simulink model "Racing_2019"  (R2017a)
settings: Solver=FixedStepDiscrete  StartTime=0.0  StopTime=Inf  FixedStep=1e-3  RelTol=1e-3  EnableMultiTasking=on
PostLoadFcn:
  | , if any(exist('dsrtsu_mdlpostloadfcn', 'file') == [2, 3, 6]), try dsrtsu_mdlpostloadfcn('Execute', bdroot); catch fprintf('Error in PostLoadFcn (dsrtsu_mdlpostloadfcn) for model "%s":\n %s\n', bdroot, lasterr); end, end,
undefined symbols (not defined in the file): Accu_Fans_Enable, Accu_Fans_ON, Accu_Fans_PWM, APPS_Bypass, APPS_Value, AUX_Error_Time, Batt_Temp_High_Threshold, Batt_Temp_Low_Threshold, BMS_Error_Time, BMS_Reset, BMS_Reset_Enable, BMS_Status_Bypass, Brake_Plausibility_Threshold, Brake_Threshold, Brakelight_Test, Braking_Torque, BSPD_State_Bypass, Buzzer, Buzzer_Silent, Buzzer_Test, Calibrate, CAN_Rx_FMEA_Enable, CAN_Status_FMEA_Enable, CAN_Tx_FMEA_Enable, Car_Reset, Car_Reset_Enable, Dash_Fan_PWM, DiscIntNeverNeededParam, DRS_Enable, DRS_PWM_OFF, DRS_PWM_ON, ED_Enable, ED_On, Eject_USB, Enable_Kill, Enable_LED_Test, Fans_Left_Enable, Fans_Left_ON, Fans_Left_PWM, Fans_Right_Enable, Fans_Right_ON, Fans_Right_PWM, I_MAX, IGBT_Temp_High_Threshold, IGBT_Temp_Low_Threshold, Inverter_CAN_Tx_Enable, Inverter_Frequency, KW_Max_Regen_Reset, KW_Max_Reset, LV_DCDC_Temp_High_Threshold, LV_DCDC_Temp_Low_Threshold, magnitude, Plausibility_Bypass, Power_Limiter_Killswitch, Power_Target_kW, Pump_Left_Enable, Pump_Left_ON, Pump_Right_Enable, Pump_Right_ON, Pump_Signal_Left ... (+13)
libraries: rtiusbflightreclib x206, simulink x153, rtican x52, powerlib_meascontrol x47, simulink_extras x17, rti1401lib_adc_type4 x6, rti1401lib_dio_type4 x3, rti1401lib_II_base x1
(part 9 of 23)

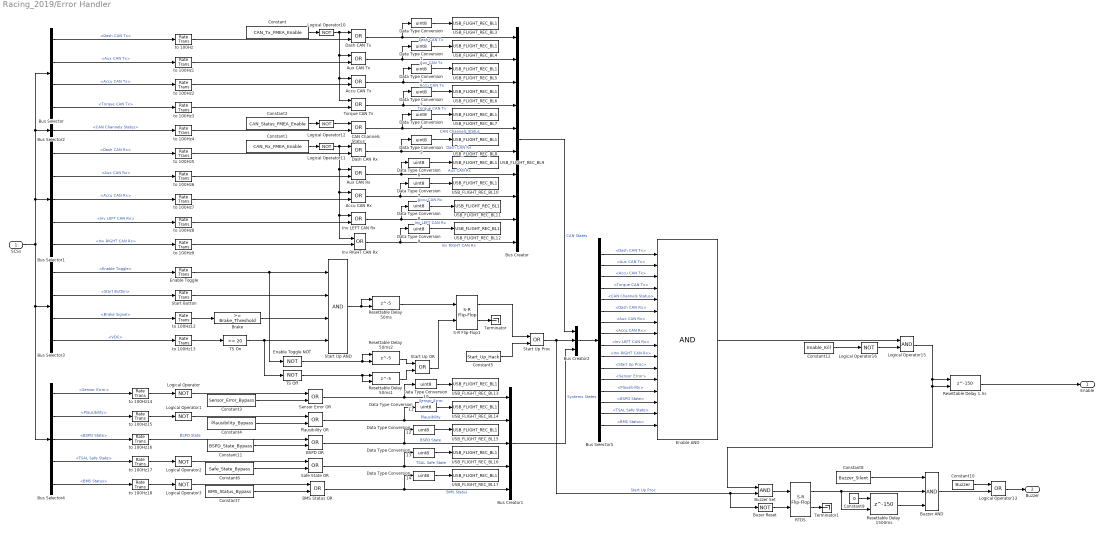
== system Racing_2019/Error Handler ==
  SCSs : Inport
  Accu CAN Rx : Logic  Operator=OR  AllPortsSameDT=off  OutDataTypeStr=boolean
  Accu CAN Tx : Logic  Operator=OR  AllPortsSameDT=off  OutDataTypeStr=boolean
  Aux CAN Rx : Logic  Operator=OR  AllPortsSameDT=off  OutDataTypeStr=boolean
  Aux CAN Tx : Logic  Operator=OR  AllPortsSameDT=off  OutDataTypeStr=boolean
  BMS Status OR : Logic  Operator=OR  AllPortsSameDT=off  OutDataTypeStr=boolean
  BSPD OR : Logic  Operator=OR  AllPortsSameDT=off  OutDataTypeStr=boolean
  Brake : simulink/Logic and Bit Operations/Compare To Constant  relop=>=  const=Brake_Threshold  OutDataTypeStr=boolean
  Bus Creator : BusCreator  Inputs='Dash CAN Tx','Aux CAN Tx','Accu CAN Tx','Torque CAN Tx','CAN Channels Status','Dash CAN Rx','Aux CAN Rx','Accu CAN Rx','Inv LEFT CAN Rx','Inv RIGHT CAN Rx'
  Bus Creator1 : BusCreator  Inputs='Sensor Error','Plausibility','BSPD State','TSAL Safe State','BMS Status'
  Bus Creator2 : BusCreator  Inputs=3
  Bus Selector : BusSelector  OutputSignals=Error & Feedback.CAN Tx Feedback.Dash CAN Tx,Error & Feedback.CAN Tx Feedback.Aux CAN Tx,Error & Feedback.CAN Tx Feedback.Accu CAN Tx,Error & Feedback.CAN Tx Feedback.Torque CAN Tx
  Bus Selector1 : BusSelector  OutputSignals=Inputs.from Dashboard.Dash CAN Rx,Inputs.from Aux.Aux CAN Rx,Inputs.from Accu.Accu CAN Rx,Inputs.from Inv LEFT.Inv LEFT CAN Rx,Inputs.from Inv RIGHT.Inv RIGHT CAN Rx
  Bus Selector2 : BusSelector  OutputSignals=Inputs.CAN Channels Status
  Bus Selector3 : BusSelector  OutputSignals=Inputs.from Dashboard.Enable Toggle,Inputs.from Dashboard.Start Button,Inputs.from Dashboard.Brake Signal,Inputs.from Gen Inputs.VDC
  Bus Selector4 : BusSelector  OutputSignals=Error & Feedback.Sensor Error,Error & Feedback.Plausibility,Inputs.from Aux.BSPD State,Inputs.from Aux.TSAL Safe State,Inputs.from Accu.BMS Status
  Bus Selector5 : BusSelector  OutputSignals=CAN States.Dash CAN Tx,CAN States.Aux CAN Tx,CAN States.Accu CAN Tx,CAN States.Torque CAN Tx,CAN States.CAN Channels Status,CAN States.Dash CAN Rx,CAN States.Aux CAN Rx,CAN States.Accu CAN Rx,CAN States.Inv LEFT CAN Rx,CAN States.Inv RIGHT CAN Rx,Start Up Proc,Systems States.Sensor Error,Systems States.Plausibility,Systems States.BSPD State,Systems States.TSAL Safe State,Systems States.BMS Status
  Buzer Reset : Logic  Operator=NOT  AllPortsSameDT=off  OutDataTypeStr=boolean
  Buzzer AND : Logic  Inputs=3  AllPortsSameDT=off  OutDataTypeStr=boolean
  Buzzer Set : Logic  AllPortsSameDT=off  OutDataTypeStr=boolean
  CAN Channels Status : Logic  Operator=OR  AllPortsSameDT=off  OutDataTypeStr=boolean
  Constant : Constant  Value=CAN_Tx_FMEA_Enable
  Constant1 : Constant  Value=CAN_Rx_FMEA_Enable
  Constant10 : Constant  Value=Buzzer
  Constant11 : Constant  Value=BSPD_State_Bypass
  Constant12 : Constant  Value=Enable_Kill
  Constant2 : Constant  Value=CAN_Status_FMEA_Enable
  Constant3 : Constant  Value=Sensor_Error_Bypass
  Constant4 : Constant  Value=Plausibility_Bypass
  Constant5 : Constant  Value=Start_Up_Hack
  Constant6 : Constant  Value=Safe_State_Bypass
  Constant7 : Constant  Value=BMS_Status_Bypass
  Constant8 : Constant  Value=Buzzer_Silent
  Constant9 : Constant  Value=0
  Dash CAN Rx : Logic  Operator=OR  AllPortsSameDT=off  OutDataTypeStr=boolean
  Dash CAN Tx : Logic  Operator=OR  AllPortsSameDT=off  OutDataTypeStr=boolean
  Data Type Conversion{,1..14} (15 alike) : DataTypeConversion  OutDataTypeStr=uint8
  Enable AND : Logic  Inputs=16  AllPortsSameDT=off  OutDataTypeStr=boolean
  Enable Toggle : RateTransition  OutPortSampleTime=0.01
  Enable Toggle NOT : Logic  Operator=NOT  AllPortsSameDT=off  OutDataTypeStr=boolean
  Inv LEFT CAN Rx : Logic  Operator=OR  AllPortsSameDT=off  OutDataTypeStr=boolean
  Inv RIGHT CAN Rx : Logic  Operator=OR  AllPortsSameDT=off  OutDataTypeStr=boolean
  Logical Operator{,1..3,10..12,16} (8 alike) : Logic  Operator=NOT  AllPortsSameDT=off  OutDataTypeStr=boolean
  Logical Operator13 : Logic  Operator=OR  AllPortsSameDT=off  OutDataTypeStr=boolean
  Logical Operator15 : Logic  AllPortsSameDT=off  OutDataTypeStr=boolean
  Plausibility OR : Logic  Operator=OR  AllPortsSameDT=off  OutDataTypeStr=boolean
  RTDS : simulink_extras/Flip Flops/S-R Flip-Flop  initial_condition=0
  Resettable Delay 1.5s : Delay  DelayLength=150  ExternalReset=Falling
      settings: InputPortMap=u0,r5
  Resettable Delay 1500ms : Delay  DelayLength=150  InitialCondition=1  ExternalReset=Rising
      settings: InputPortMap=u0,r5
  Resettable Delay 50ms : Delay  DelayLength=5  ExternalReset=Falling
      settings: InputPortMap=u0,r5
  Resettable Delay 50ms1 : Delay  DelayLength=5  InitialCondition=1  ExternalReset=Rising
      settings: InputPortMap=u0,r5
  Resettable Delay 50ms2 : Delay  DelayLength=5  InitialCondition=1  ExternalReset=Rising
      settings: InputPortMap=u0,r5
  S-R Flip-Flop1 : simulink_extras/Flip Flops/S-R Flip-Flop  initial_condition=0
  Safe State OR : Logic  Operator=OR  AllPortsSameDT=off  OutDataTypeStr=boolean
  "Sensor Error OR " : Logic  Operator=OR  AllPortsSameDT=off  OutDataTypeStr=boolean
  Start Button : RateTransition  OutPortSampleTime=0.01
  Start Up AND : Logic  Inputs=4  AllPortsSameDT=off  OutDataTypeStr=boolean
  Start Up OR : Logic  Operator=OR  AllPortsSameDT=off  OutDataTypeStr=boolean
  Start Up Proc : Logic  Operator=OR  AllPortsSameDT=off  OutDataTypeStr=boolean
  TS Off : Logic  Operator=NOT  AllPortsSameDT=off  OutDataTypeStr=boolean
  TS On : simulink/Logic and Bit Operations/Compare To Constant  relop=>=  const=20  OutDataTypeStr=boolean
  Terminator : Terminator
  Terminator1 : Terminator
  Torque CAN Tx : Logic  Operator=OR  AllPortsSameDT=off  OutDataTypeStr=boolean
  USB_FLIGHT_REC_BL10 : rtiusbflightreclib/USB_FLIGHT_REC_BL1  VarName=ENABLE_Accu_CAN_Rx  DataType=UInt8  SampleTime=-1  TLCFileName=rtiusbflightrecwrite  Reserved1=[]  Reserved2=[]  Reserved3=[]  Reserved4=[]  DSProperties=struct('RTI',struct('Version',uint32(3),'BlockType',struct('isSLSource',uint8(0),'isSLSink',uint8(1),'isHWSource',uint8(0),'isHWSink',uint8(0),'isSetup',uint8(0),'isInline',uint8(1),'isNonInline',uint8(0),'isInterrupt',uint8(0),'isChannelwise',uint8(0)),'IOBoardType',{{'DSUSB','FLIGHTREC'}},'UnitType','FLIGHTREC','Identifier','WRITE','DialogType','SL','BlockSet','RTIUSBFLIGHTREC','SlaveProcessor','NONE'))  RTIBlockInterface=struct('InputPortsActive',1,'InputPortsWidth',int32(1),'InputPortsDataType',{{'SS_UINT8'}},'BlockDisplay',{{['Write to\nUSB Flight Recorder'],'center'}},'IconTransparency','off','InitLevel',3,'BlockName',struct('Token',{{'USB_FLIGHT_REC_BL1'}}),'MaskDescription',['Write input to the Flight Recorder. Recorded data can be referenced by the specified variable.'],'SampleTime',{{-1}})  RTIBlockParameters=struct('VarName',{{'ENABLE_Accu_CAN_Rx','OFF',[]}},'DataType',{{'UInt8','OFF',[]}},'SampleTime',{{-1,'OFF',[]}},'TLCFileName',{{'rtiusbflightrecwrite','OFF',[]}})  RTISFcnParameters=struct('VarName','char','DataType','char','SampleTime','double','TLCFileName','char')  RTIBlockParaDefault=struct('VarName','Var1','DataType','Single','SampleTime',-1,'TLCFileName','rtiusbflightrecwrite')
      settings: SourceProductName=dSPACE RTI USB Flight Rec Blockset
  USB_FLIGHT_REC_BL11 : rtiusbflightreclib/USB_FLIGHT_REC_BL1  VarName=ENABLE_Inv_LEFT_CAN_Rx  DataType=UInt8  SampleTime=-1  TLCFileName=rtiusbflightrecwrite  Reserved1=[]  Reserved2=[]  Reserved3=[]  Reserved4=[]  DSProperties=struct('RTI',struct('Version',uint32(3),'BlockType',struct('isSLSource',uint8(0),'isSLSink',uint8(1),'isHWSource',uint8(0),'isHWSink',uint8(0),'isSetup',uint8(0),'isInline',uint8(1),'isNonInline',uint8(0),'isInterrupt',uint8(0),'isChannelwise',uint8(0)),'IOBoardType',{{'DSUSB','FLIGHTREC'}},'UnitType','FLIGHTREC','Identifier','WRITE','DialogType','SL','BlockSet','RTIUSBFLIGHTREC','SlaveProcessor','NONE'))  RTIBlockInterface=struct('InputPortsActive',1,'InputPortsWidth',int32(1),'InputPortsDataType',{{'SS_UINT8'}},'BlockDisplay',{{['Write to\nUSB Flight Recorder'],'center'}},'IconTransparency','off','InitLevel',3,'BlockName',struct('Token',{{'USB_FLIGHT_REC_BL1'}}),'MaskDescription',['Write input to the Flight Recorder. Recorded data can be referenced by the specified variable.'],'SampleTime',{{-1}})  RTIBlockParameters=struct('VarName',{{'ENABLE_Inv_LEFT_CAN_Rx','OFF',[]}},'DataType',{{'UInt8','OFF',[]}},'SampleTime',{{-1,'OFF',[]}},'TLCFileName',{{'rtiusbflightrecwrite','OFF',[]}})  RTISFcnParameters=struct('VarName','char','DataType','char','SampleTime','double','TLCFileName','char')  RTIBlockParaDefault=struct('VarName','Var1','DataType','Single','SampleTime',-1,'TLCFileName','rtiusbflightrecwrite')
      settings: SourceProductName=dSPACE RTI USB Flight Rec Blockset
  USB_FLIGHT_REC_BL12 : rtiusbflightreclib/USB_FLIGHT_REC_BL1  VarName=ENABLE_Inv_RIGHT_CAN_Rx  DataType=UInt8  SampleTime=-1  TLCFileName=rtiusbflightrecwrite  Reserved1=[]  Reserved2=[]  Reserved3=[]  Reserved4=[]  DSProperties=struct('RTI',struct('Version',uint32(3),'BlockType',struct('isSLSource',uint8(0),'isSLSink',uint8(1),'isHWSource',uint8(0),'isHWSink',uint8(0),'isSetup',uint8(0),'isInline',uint8(1),'isNonInline',uint8(0),'isInterrupt',uint8(0),'isChannelwise',uint8(0)),'IOBoardType',{{'DSUSB','FLIGHTREC'}},'UnitType','FLIGHTREC','Identifier','WRITE','DialogType','SL','BlockSet','RTIUSBFLIGHTREC','SlaveProcessor','NONE'))  RTIBlockInterface=struct('InputPortsActive',1,'InputPortsWidth',int32(1),'InputPortsDataType',{{'SS_UINT8'}},'BlockDisplay',{{['Write to\nUSB Flight Recorder'],'center'}},'IconTransparency','off','InitLevel',3,'BlockName',struct('Token',{{'USB_FLIGHT_REC_BL1'}}),'MaskDescription',['Write input to the Flight Recorder. Recorded data can be referenced by the specified variable.'],'SampleTime',{{-1}})  RTIBlockParameters=struct('VarName',{{'ENABLE_Inv_RIGHT_CAN_Rx','OFF',[]}},'DataType',{{'UInt8','OFF',[]}},'SampleTime',{{-1,'OFF',[]}},'TLCFileName',{{'rtiusbflightrecwrite','OFF',[]}})  RTISFcnParameters=struct('VarName','char','DataType','char','SampleTime','double','TLCFileName','char')  RTIBlockParaDefault=struct('VarName','Var1','DataType','Single','SampleTime',-1,'TLCFileName','rtiusbflightrecwrite')
      settings: SourceProductName=dSPACE RTI USB Flight Rec Blockset
  USB_FLIGHT_REC_BL13 : rtiusbflightreclib/USB_FLIGHT_REC_BL1  VarName=ENABLE_Sensor_Error  DataType=UInt8  SampleTime=-1  TLCFileName=rtiusbflightrecwrite  Reserved1=[]  Reserved2=[]  Reserved3=[]  Reserved4=[]  DSProperties=struct('RTI',struct('Version',uint32(3),'BlockType',struct('isSLSource',uint8(0),'isSLSink',uint8(1),'isHWSource',uint8(0),'isHWSink',uint8(0),'isSetup',uint8(0),'isInline',uint8(1),'isNonInline',uint8(0),'isInterrupt',uint8(0),'isChannelwise',uint8(0)),'IOBoardType',{{'DSUSB','FLIGHTREC'}},'UnitType','FLIGHTREC','Identifier','WRITE','DialogType','SL','BlockSet','RTIUSBFLIGHTREC','SlaveProcessor','NONE'))  RTIBlockInterface=struct('InputPortsActive',1,'InputPortsWidth',int32(1),'InputPortsDataType',{{'SS_UINT8'}},'BlockDisplay',{{['Write to\nUSB Flight Recorder'],'center'}},'IconTransparency','off','InitLevel',3,'BlockName',struct('Token',{{'USB_FLIGHT_REC_BL1'}}),'MaskDescription',['Write input to the Flight Recorder. Recorded data can be referenced by the specified variable.'],'SampleTime',{{-1}})  RTIBlockParameters=struct('VarName',{{'ENABLE_Sensor_Error','OFF',[]}},'DataType',{{'UInt8','OFF',[]}},'SampleTime',{{-1,'OFF',[]}},'TLCFileName',{{'rtiusbflightrecwrite','OFF',[]}})  RTISFcnParameters=struct('VarName','char','DataType','char','SampleTime','double','TLCFileName','char')  RTIBlockParaDefault=struct('VarName','Var1','DataType','Single','SampleTime',-1,'TLCFileName','rtiusbflightrecwrite')
      settings: SourceProductName=dSPACE RTI USB Flight Rec Blockset
  USB_FLIGHT_REC_BL14 : rtiusbflightreclib/USB_FLIGHT_REC_BL1  VarName=ENABLE_Plausibility  DataType=UInt8  SampleTime=-1  TLCFileName=rtiusbflightrecwrite  Reserved1=[]  Reserved2=[]  Reserved3=[]  Reserved4=[]  DSProperties=struct('RTI',struct('Version',uint32(3),'BlockType',struct('isSLSource',uint8(0),'isSLSink',uint8(1),'isHWSource',uint8(0),'isHWSink',uint8(0),'isSetup',uint8(0),'isInline',uint8(1),'isNonInline',uint8(0),'isInterrupt',uint8(0),'isChannelwise',uint8(0)),'IOBoardType',{{'DSUSB','FLIGHTREC'}},'UnitType','FLIGHTREC','Identifier','WRITE','DialogType','SL','BlockSet','RTIUSBFLIGHTREC','SlaveProcessor','NONE'))  RTIBlockInterface=struct('InputPortsActive',1,'InputPortsWidth',int32(1),'InputPortsDataType',{{'SS_UINT8'}},'BlockDisplay',{{['Write to\nUSB Flight Recorder'],'center'}},'IconTransparency','off','InitLevel',3,'BlockName',struct('Token',{{'USB_FLIGHT_REC_BL1'}}),'MaskDescription',['Write input to the Flight Recorder. Recorded data can be referenced by the specified variable.'],'SampleTime',{{-1}})  RTIBlockParameters=struct('VarName',{{'ENABLE_Plausibility','OFF',[]}},'DataType',{{'UInt8','OFF',[]}},'SampleTime',{{-1,'OFF',[]}},'TLCFileName',{{'rtiusbflightrecwrite','OFF',[]}})  RTISFcnParameters=struct('VarName','char','DataType','char','SampleTime','double','TLCFileName','char')  RTIBlockParaDefault=struct('VarName','Var1','DataType','Single','SampleTime',-1,'TLCFileName','rtiusbflightrecwrite')
      settings: SourceProductName=dSPACE RTI USB Flight Rec Blockset
  USB_FLIGHT_REC_BL15 : rtiusbflightreclib/USB_FLIGHT_REC_BL1  VarName=ENABLE_BSPD_State  DataType=UInt8  SampleTime=-1  TLCFileName=rtiusbflightrecwrite  Reserved1=[]  Reserved2=[]  Reserved3=[]  Reserved4=[]  DSProperties=struct('RTI',struct('Version',uint32(3),'BlockType',struct('isSLSource',uint8(0),'isSLSink',uint8(1),'isHWSource',uint8(0),'isHWSink',uint8(0),'isSetup',uint8(0),'isInline',uint8(1),'isNonInline',uint8(0),'isInterrupt',uint8(0),'isChannelwise',uint8(0)),'IOBoardType',{{'DSUSB','FLIGHTREC'}},'UnitType','FLIGHTREC','Identifier','WRITE','DialogType','SL','BlockSet','RTIUSBFLIGHTREC','SlaveProcessor','NONE'))  RTIBlockInterface=struct('InputPortsActive',1,'InputPortsWidth',int32(1),'InputPortsDataType',{{'SS_UINT8'}},'BlockDisplay',{{['Write to\nUSB Flight Recorder'],'center'}},'IconTransparency','off','InitLevel',3,'BlockName',struct('Token',{{'USB_FLIGHT_REC_BL1'}}),'MaskDescription',['Write input to the Flight Recorder. Recorded data can be referenced by the specified variable.'],'SampleTime',{{-1}})  RTIBlockParameters=struct('VarName',{{'ENABLE_BSPD_State','OFF',[]}},'DataType',{{'UInt8','OFF',[]}},'SampleTime',{{-1,'OFF',[]}},'TLCFileName',{{'rtiusbflightrecwrite','OFF',[]}})  RTISFcnParameters=struct('VarName','char','DataType','char','SampleTime','double','TLCFileName','char')  RTIBlockParaDefault=struct('VarName','Var1','DataType','Single','SampleTime',-1,'TLCFileName','rtiusbflightrecwrite')
      settings: SourceProductName=dSPACE RTI USB Flight Rec Blockset
  USB_FLIGHT_REC_BL16 : rtiusbflightreclib/USB_FLIGHT_REC_BL1  VarName=ENABLE_TSAL_Safe_State  DataType=UInt8  SampleTime=-1  TLCFileName=rtiusbflightrecwrite  Reserved1=[]  Reserved2=[]  Reserved3=[]  Reserved4=[]  DSProperties=struct('RTI',struct('Version',uint32(3),'BlockType',struct('isSLSource',uint8(0),'isSLSink',uint8(1),'isHWSource',uint8(0),'isHWSink',uint8(0),'isSetup',uint8(0),'isInline',uint8(1),'isNonInline',uint8(0),'isInterrupt',uint8(0),'isChannelwise',uint8(0)),'IOBoardType',{{'DSUSB','FLIGHTREC'}},'UnitType','FLIGHTREC','Identifier','WRITE','DialogType','SL','BlockSet','RTIUSBFLIGHTREC','SlaveProcessor','NONE'))  RTIBlockInterface=struct('InputPortsActive',1,'InputPortsWidth',int32(1),'InputPortsDataType',{{'SS_UINT8'}},'BlockDisplay',{{['Write to\nUSB Flight Recorder'],'center'}},'IconTransparency','off','InitLevel',3,'BlockName',struct('Token',{{'USB_FLIGHT_REC_BL1'}}),'MaskDescription',['Write input to the Flight Recorder. Recorded data can be referenced by the specified variable.'],'SampleTime',{{-1}})  RTIBlockParameters=struct('VarName',{{'ENABLE_TSAL_Safe_State','OFF',[]}},'DataType',{{'UInt8','OFF',[]}},'SampleTime',{{-1,'OFF',[]}},'TLCFileName',{{'rtiusbflightrecwrite','OFF',[]}})  RTISFcnParameters=struct('VarName','char','DataType','char','SampleTime','double','TLCFileName','char')  RTIBlockParaDefault=struct('VarName','Var1','DataType','Single','SampleTime',-1,'TLCFileName','rtiusbflightrecwrite')
      settings: SourceProductName=dSPACE RTI USB Flight Rec Blockset
  USB_FLIGHT_REC_BL17 : rtiusbflightreclib/USB_FLIGHT_REC_BL1  VarName=ENABLE_BMS_Status  DataType=UInt8  SampleTime=-1  TLCFileName=rtiusbflightrecwrite  Reserved1=[]  Reserved2=[]  Reserved3=[]  Reserved4=[]  DSProperties=struct('RTI',struct('Version',uint32(3),'BlockType',struct('isSLSource',uint8(0),'isSLSink',uint8(1),'isHWSource',uint8(0),'isHWSink',uint8(0),'isSetup',uint8(0),'isInline',uint8(1),'isNonInline',uint8(0),'isInterrupt',uint8(0),'isChannelwise',uint8(0)),'IOBoardType',{{'DSUSB','FLIGHTREC'}},'UnitType','FLIGHTREC','Identifier','WRITE','DialogType','SL','BlockSet','RTIUSBFLIGHTREC','SlaveProcessor','NONE'))  RTIBlockInterface=struct('InputPortsActive',1,'InputPortsWidth',int32(1),'InputPortsDataType',{{'SS_UINT8'}},'BlockDisplay',{{['Write to\nUSB Flight Recorder'],'center'}},'IconTransparency','off','InitLevel',3,'BlockName',struct('Token',{{'USB_FLIGHT_REC_BL1'}}),'MaskDescription',['Write input to the Flight Recorder. Recorded data can be referenced by the specified variable.'],'SampleTime',{{-1}})  RTIBlockParameters=struct('VarName',{{'ENABLE_BMS_Status','OFF',[]}},'DataType',{{'UInt8','OFF',[]}},'SampleTime',{{-1,'OFF',[]}},'TLCFileName',{{'rtiusbflightrecwrite','OFF',[]}})  RTISFcnParameters=struct('VarName','char','DataType','char','SampleTime','double','TLCFileName','char')  RTIBlockParaDefault=struct('VarName','Var1','DataType','Single','SampleTime',-1,'TLCFileName','rtiusbflightrecwrite')
      settings: SourceProductName=dSPACE RTI USB Flight Rec Blockset
  USB_FLIGHT_REC_BL3 : rtiusbflightreclib/USB_FLIGHT_REC_BL1  VarName=ENABLE_Dash_CAN_Tx  DataType=UInt8  SampleTime=-1  TLCFileName=rtiusbflightrecwrite  Reserved1=[]  Reserved2=[]  Reserved3=[]  Reserved4=[]  DSProperties=struct('RTI',struct('Version',uint32(3),'BlockType',struct('isSLSource',uint8(0),'isSLSink',uint8(1),'isHWSource',uint8(0),'isHWSink',uint8(0),'isSetup',uint8(0),'isInline',uint8(1),'isNonInline',uint8(0),'isInterrupt',uint8(0),'isChannelwise',uint8(0)),'IOBoardType',{{'DSUSB','FLIGHTREC'}},'UnitType','FLIGHTREC','Identifier','WRITE','DialogType','SL','BlockSet','RTIUSBFLIGHTREC','SlaveProcessor','NONE'))  RTIBlockInterface=struct('InputPortsActive',1,'InputPortsWidth',int32(1),'InputPortsDataType',{{'SS_UINT8'}},'BlockDisplay',{{['Write to\nUSB Flight Recorder'],'center'}},'IconTransparency','off','InitLevel',3,'BlockName',struct('Token',{{'USB_FLIGHT_REC_BL1'}}),'MaskDescription',['Write input to the Flight Recorder. Recorded data can be referenced by the specified variable.'],'SampleTime',{{-1}})  RTIBlockParameters=struct('VarName',{{'ENABLE_Dash_CAN_Tx','OFF',[]}},'DataType',{{'UInt8','OFF',[]}},'SampleTime',{{-1,'OFF',[]}},'TLCFileName',{{'rtiusbflightrecwrite','OFF',[]}})  RTISFcnParameters=struct('VarName','char','DataType','char','SampleTime','double','TLCFileName','char')  RTIBlockParaDefault=struct('VarName','Var1','DataType','Single','SampleTime',-1,'TLCFileName','rtiusbflightrecwrite')
      settings: SourceProductName=dSPACE RTI USB Flight Rec Blockset
  USB_FLIGHT_REC_BL4 : rtiusbflightreclib/USB_FLIGHT_REC_BL1  VarName=ENABLE_Aux_CAN_Tx  DataType=UInt8  SampleTime=-1  TLCFileName=rtiusbflightrecwrite  Reserved1=[]  Reserved2=[]  Reserved3=[]  Reserved4=[]  DSProperties=struct('RTI',struct('Version',uint32(3),'BlockType',struct('isSLSource',uint8(0),'isSLSink',uint8(1),'isHWSource',uint8(0),'isHWSink',uint8(0),'isSetup',uint8(0),'isInline',uint8(1),'isNonInline',uint8(0),'isInterrupt',uint8(0),'isChannelwise',uint8(0)),'IOBoardType',{{'DSUSB','FLIGHTREC'}},'UnitType','FLIGHTREC','Identifier','WRITE','DialogType','SL','BlockSet','RTIUSBFLIGHTREC','SlaveProcessor','NONE'))  RTIBlockInterface=struct('InputPortsActive',1,'InputPortsWidth',int32(1),'InputPortsDataType',{{'SS_UINT8'}},'BlockDisplay',{{['Write to\nUSB Flight Recorder'],'center'}},'IconTransparency','off','InitLevel',3,'BlockName',struct('Token',{{'USB_FLIGHT_REC_BL1'}}),'MaskDescription',['Write input to the Flight Recorder. Recorded data can be referenced by the specified variable.'],'SampleTime',{{-1}})  RTIBlockParameters=struct('VarName',{{'ENABLE_Aux_CAN_Tx','OFF',[]}},'DataType',{{'UInt8','OFF',[]}},'SampleTime',{{-1,'OFF',[]}},'TLCFileName',{{'rtiusbflightrecwrite','OFF',[]}})  RTISFcnParameters=struct('VarName','char','DataType','char','SampleTime','double','TLCFileName','char')  RTIBlockParaDefault=struct('VarName','Var1','DataType','Single','SampleTime',-1,'TLCFileName','rtiusbflightrecwrite')
      settings: SourceProductName=dSPACE RTI USB Flight Rec Blockset
  USB_FLIGHT_REC_BL5 : rtiusbflightreclib/USB_FLIGHT_REC_BL1  VarName=ENABLE_Accu_CAN_Tx  DataType=UInt8  SampleTime=-1  TLCFileName=rtiusbflightrecwrite  Reserved1=[]  Reserved2=[]  Reserved3=[]  Reserved4=[]  DSProperties=struct('RTI',struct('Version',uint32(3),'BlockType',struct('isSLSource',uint8(0),'isSLSink',uint8(1),'isHWSource',uint8(0),'isHWSink',uint8(0),'isSetup',uint8(0),'isInline',uint8(1),'isNonInline',uint8(0),'isInterrupt',uint8(0),'isChannelwise',uint8(0)),'IOBoardType',{{'DSUSB','FLIGHTREC'}},'UnitType','FLIGHTREC','Identifier','WRITE','DialogType','SL','BlockSet','RTIUSBFLIGHTREC','SlaveProcessor','NONE'))  RTIBlockInterface=struct('InputPortsActive',1,'InputPortsWidth',int32(1),'InputPortsDataType',{{'SS_UINT8'}},'BlockDisplay',{{['Write to\nUSB Flight Recorder'],'center'}},'IconTransparency','off','InitLevel',3,'BlockName',struct('Token',{{'USB_FLIGHT_REC_BL1'}}),'MaskDescription',['Write input to the Flight Recorder. Recorded data can be referenced by the specified variable.'],'SampleTime',{{-1}})  RTIBlockParameters=struct('VarName',{{'ENABLE_Accu_CAN_Tx','OFF',[]}},'DataType',{{'UInt8','OFF',[]}},'SampleTime',{{-1,'OFF',[]}},'TLCFileName',{{'rtiusbflightrecwrite','OFF',[]}})  RTISFcnParameters=struct('VarName','char','DataType','char','SampleTime','double','TLCFileName','char')  RTIBlockParaDefault=struct('VarName','Var1','DataType','Single','SampleTime',-1,'TLCFileName','rtiusbflightrecwrite')
      settings: SourceProductName=dSPACE RTI USB Flight Rec Blockset
  USB_FLIGHT_REC_BL6 : rtiusbflightreclib/USB_FLIGHT_REC_BL1  VarName=ENABLE_Torque_CAN_Tx  DataType=UInt8  SampleTime=-1  TLCFileName=rtiusbflightrecwrite  Reserved1=[]  Reserved2=[]  Reserved3=[]  Reserved4=[]  DSProperties=struct('RTI',struct('Version',uint32(3),'BlockType',struct('isSLSource',uint8(0),'isSLSink',uint8(1),'isHWSource',uint8(0),'isHWSink',uint8(0),'isSetup',uint8(0),'isInline',uint8(1),'isNonInline',uint8(0),'isInterrupt',uint8(0),'isChannelwise',uint8(0)),'IOBoardType',{{'DSUSB','FLIGHTREC'}},'UnitType','FLIGHTREC','Identifier','WRITE','DialogType','SL','BlockSet','RTIUSBFLIGHTREC','SlaveProcessor','NONE'))  RTIBlockInterface=struct('InputPortsActive',1,'InputPortsWidth',int32(1),'InputPortsDataType',{{'SS_UINT8'}},'BlockDisplay',{{['Write to\nUSB Flight Recorder'],'center'}},'IconTransparency','off','InitLevel',3,'BlockName',struct('Token',{{'USB_FLIGHT_REC_BL1'}}),'MaskDescription',['Write input to the Flight Recorder. Recorded data can be referenced by the specified variable.'],'SampleTime',{{-1}})  RTIBlockParameters=struct('VarName',{{'ENABLE_Torque_CAN_Tx','OFF',[]}},'DataType',{{'UInt8','OFF',[]}},'SampleTime',{{-1,'OFF',[]}},'TLCFileName',{{'rtiusbflightrecwrite','OFF',[]}})  RTISFcnParameters=struct('VarName','char','DataType','char','SampleTime','double','TLCFileName','char')  RTIBlockParaDefault=struct('VarName','Var1','DataType','Single','SampleTime',-1,'TLCFileName','rtiusbflightrecwrite')
      settings: SourceProductName=dSPACE RTI USB Flight Rec Blockset
  USB_FLIGHT_REC_BL7 : rtiusbflightreclib/USB_FLIGHT_REC_BL1  VarName=ENABLE_CAN_Status  DataType=UInt8  SampleTime=-1  TLCFileName=rtiusbflightrecwrite  Reserved1=[]  Reserved2=[]  Reserved3=[]  Reserved4=[]  DSProperties=struct('RTI',struct('Version',uint32(3),'BlockType',struct('isSLSource',uint8(0),'isSLSink',uint8(1),'isHWSource',uint8(0),'isHWSink',uint8(0),'isSetup',uint8(0),'isInline',uint8(1),'isNonInline',uint8(0),'isInterrupt',uint8(0),'isChannelwise',uint8(0)),'IOBoardType',{{'DSUSB','FLIGHTREC'}},'UnitType','FLIGHTREC','Identifier','WRITE','DialogType','SL','BlockSet','RTIUSBFLIGHTREC','SlaveProcessor','NONE'))  RTIBlockInterface=struct('InputPortsActive',1,'InputPortsWidth',int32(1),'InputPortsDataType',{{'SS_UINT8'}},'BlockDisplay',{{['Write to\nUSB Flight Recorder'],'center'}},'IconTransparency','off','InitLevel',3,'BlockName',struct('Token',{{'USB_FLIGHT_REC_BL1'}}),'MaskDescription',['Write input to the Flight Recorder. Recorded data can be referenced by the specified variable.'],'SampleTime',{{-1}})  RTIBlockParameters=struct('VarName',{{'ENABLE_CAN_Status','OFF',[]}},'DataType',{{'UInt8','OFF',[]}},'SampleTime',{{-1,'OFF',[]}},'TLCFileName',{{'rtiusbflightrecwrite','OFF',[]}})  RTISFcnParameters=struct('VarName','char','DataType','char','SampleTime','double','TLCFileName','char')  RTIBlockParaDefault=struct('VarName','Var1','DataType','Single','SampleTime',-1,'TLCFileName','rtiusbflightrecwrite')
      settings: SourceProductName=dSPACE RTI USB Flight Rec Blockset
  USB_FLIGHT_REC_BL8 : rtiusbflightreclib/USB_FLIGHT_REC_BL1  VarName=ENABLE_Dash_CAN_Rx  DataType=UInt8  SampleTime=-1  TLCFileName=rtiusbflightrecwrite  Reserved1=[]  Reserved2=[]  Reserved3=[]  Reserved4=[]  DSProperties=struct('RTI',struct('Version',uint32(3),'BlockType',struct('isSLSource',uint8(0),'isSLSink',uint8(1),'isHWSource',uint8(0),'isHWSink',uint8(0),'isSetup',uint8(0),'isInline',uint8(1),'isNonInline',uint8(0),'isInterrupt',uint8(0),'isChannelwise',uint8(0)),'IOBoardType',{{'DSUSB','FLIGHTREC'}},'UnitType','FLIGHTREC','Identifier','WRITE','DialogType','SL','BlockSet','RTIUSBFLIGHTREC','SlaveProcessor','NONE'))  RTIBlockInterface=struct('InputPortsActive',1,'InputPortsWidth',int32(1),'InputPortsDataType',{{'SS_UINT8'}},'BlockDisplay',{{['Write to\nUSB Flight Recorder'],'center'}},'IconTransparency','off','InitLevel',3,'BlockName',struct('Token',{{'USB_FLIGHT_REC_BL1'}}),'MaskDescription',['Write input to the Flight Recorder. Recorded data can be referenced by the specified variable.'],'SampleTime',{{-1}})  RTIBlockParameters=struct('VarName',{{'ENABLE_Dash_CAN_Rx','OFF',[]}},'DataType',{{'UInt8','OFF',[]}},'SampleTime',{{-1,'OFF',[]}},'TLCFileName',{{'rtiusbflightrecwrite','OFF',[]}})  RTISFcnParameters=struct('VarName','char','DataType','char','SampleTime','double','TLCFileName','char')  RTIBlockParaDefault=struct('VarName','Var1','DataType','Single','SampleTime',-1,'TLCFileName','rtiusbflightrecwrite')
      settings: SourceProductName=dSPACE RTI USB Flight Rec Blockset
  USB_FLIGHT_REC_BL9 : rtiusbflightreclib/USB_FLIGHT_REC_BL1  VarName=ENABLE_Aux_CAN_Rx  DataType=UInt8  SampleTime=-1  TLCFileName=rtiusbflightrecwrite  Reserved1=[]  Reserved2=[]  Reserved3=[]  Reserved4=[]  DSProperties=struct('RTI',struct('Version',uint32(3),'BlockType',struct('isSLSource',uint8(0),'isSLSink',uint8(1),'isHWSource',uint8(0),'isHWSink',uint8(0),'isSetup',uint8(0),'isInline',uint8(1),'isNonInline',uint8(0),'isInterrupt',uint8(0),'isChannelwise',uint8(0)),'IOBoardType',{{'DSUSB','FLIGHTREC'}},'UnitType','FLIGHTREC','Identifier','WRITE','DialogType','SL','BlockSet','RTIUSBFLIGHTREC','SlaveProcessor','NONE'))  RTIBlockInterface=struct('InputPortsActive',1,'InputPortsWidth',int32(1),'InputPortsDataType',{{'SS_UINT8'}},'BlockDisplay',{{['Write to\nUSB Flight Recorder'],'center'}},'IconTransparency','off','InitLevel',3,'BlockName',struct('Token',{{'USB_FLIGHT_REC_BL1'}}),'MaskDescription',['Write input to the Flight Recorder. Recorded data can be referenced by the specified variable.'],'SampleTime',{{-1}})  RTIBlockParameters=struct('VarName',{{'ENABLE_Aux_CAN_Rx','OFF',[]}},'DataType',{{'UInt8','OFF',[]}},'SampleTime',{{-1,'OFF',[]}},'TLCFileName',{{'rtiusbflightrecwrite','OFF',[]}})  RTISFcnParameters=struct('VarName','char','DataType','char','SampleTime','double','TLCFileName','char')  RTIBlockParaDefault=struct('VarName','Var1','DataType','Single','SampleTime',-1,'TLCFileName','rtiusbflightrecwrite')
      settings: SourceProductName=dSPACE RTI USB Flight Rec Blockset
  to 100Hz{,1..9,12..18} (17 alike) : RateTransition  OutPortSampleTime=0.01
  Enable : Outport
  Buzzer : Outport  Port=2
  wires:
  SCSs/1 -> Bus Selector/1, Bus Selector2/1, Bus Selector1/1, Bus Selector4/1, Bus Selector3/1
  to 100Hz/1 -> Dash CAN Tx/2
  to 100Hz1/1 -> Aux CAN Tx/2
  to 100Hz2/1 -> Accu CAN Tx/2
  to 100Hz3/1 -> Torque CAN Tx/2
  to 100Hz4/1 -> CAN Channels Status/2
  to 100Hz5/1 -> Dash CAN Rx/2
  to 100Hz6/1 -> Aux CAN Rx/2
  to 100Hz7/1 -> Accu CAN Rx/2
  to 100Hz8/1 -> Inv LEFT CAN Rx/2
  to 100Hz9/1 -> Inv RIGHT CAN Rx/2
  Constant/1 -> Logical Operator10/1
  Constant1/1 -> Logical Operator11/1
  Constant2/1 -> Logical Operator12/1
  Logical Operator12/1 -> CAN Channels Status/1
  to 100Hz12/1 -> Brake/1
  to 100Hz13/1 -> TS On/1
  Enable Toggle/1 -> Start Up AND/1, Enable Toggle NOT/1
  Start Button/1 -> Start Up AND/2
  Brake/1 -> Start Up AND/3
  TS On/1 -> TS Off/1, Start Up AND/4
  Start Up AND/1 -> Resettable Delay 50ms/1, Resettable Delay 50ms/2
  Resettable Delay 50ms/1 -> S-R Flip-Flop1/1
  S-R Flip-Flop1/2 -> Terminator/1
  TS Off/1 -> Resettable Delay 50ms1/2, Resettable Delay 50ms1/1
  to 100Hz14/1 -> Logical Operator/1
  Constant3/1 -> "Sensor Error OR "/2
  Constant4/1 -> Plausibility OR/2
  to 100Hz15/1 -> Logical Operator1/1
  Constant6/1 -> Safe State OR/2
  to 100Hz17/1 -> Logical Operator2/1
  Constant7/1 -> BMS Status OR/2
  to 100Hz18/1 -> Logical Operator3/1
  S-R Flip-Flop1/1 -> Start Up Proc/1
  Start Up Proc/1 -> Bus Creator2/2, Buzer Reset/1, Buzzer Set/2  "Start Up Proc"
  Constant5/1 -> Start Up Proc/2
  Enable Toggle NOT/1 -> Resettable Delay 50ms2/1, Resettable Delay 50ms2/2
  Resettable Delay 50ms2/1 -> Start Up OR/1
  Resettable Delay 50ms1/1 -> Start Up OR/2
  Start Up OR/1 -> S-R Flip-Flop1/2
  Buzzer Set/1 -> RTDS/1
  Buzer Reset/1 -> RTDS/2
  Resettable Delay 1.5s/1 -> Enable/1
  RTDS/1 -> Resettable Delay 1500ms/2, Buzzer AND/2
  Constant8/1 -> Buzzer AND/1
  Constant9/1 -> Resettable Delay 1500ms/1
  Resettable Delay 1500ms/1 -> Buzzer AND/3
  Buzzer AND/1 -> Logical Operator13/2
  Constant10/1 -> Logical Operator13/1
  Logical Operator13/1 -> Buzzer/1
  Bus Selector/1 -> to 100Hz/1  "<Dash CAN Tx>"
  Bus Selector/2 -> to 100Hz1/1  "<Aux CAN Tx>"
  Bus Selector/3 -> to 100Hz2/1  "<Accu CAN Tx>"
  Bus Selector/4 -> to 100Hz3/1  "<Torque CAN Tx>"
  Bus Selector2/1 -> to 100Hz4/1  "<CAN Channels Status>"
  Bus Selector1/1 -> to 100Hz5/1  "<Dash CAN Rx>"
  Bus Selector1/2 -> to 100Hz6/1  "<Aux CAN Rx>"
  Bus Selector1/3 -> to 100Hz7/1  "<Accu CAN Rx>"
  Bus Selector1/4 -> to 100Hz8/1  "<Inv LEFT CAN Rx>"
  Bus Selector1/5 -> to 100Hz9/1  "<Inv RIGHT CAN Rx>"
  Bus Selector3/1 -> Enable Toggle/1  "<Enable Toggle>"
  Bus Selector3/2 -> Start Button/1  "<Start Button>"
  Bus Selector3/3 -> to 100Hz12/1  "<Brake Signal>"
  Bus Selector3/4 -> to 100Hz13/1  "<VDC>"
  Bus Selector4/1 -> to 100Hz14/1  "<Sensor Error>"
  Bus Selector4/2 -> to 100Hz15/1  "<Plausibility>"
  Bus Selector4/3 -> to 100Hz16/1  "<BSPD State>"
  Bus Selector4/4 -> to 100Hz17/1  "<TSAL Safe State>"
  Bus Selector4/5 -> to 100Hz18/1  "<BMS Status>"
  RTDS/2 -> Terminator1/1
  Dash CAN Tx/1 -> Bus Creator/1, Data Type Conversion/1  "Dash CAN Tx"
  Aux CAN Tx/1 -> Bus Creator/2, Data Type Conversion1/1  "Aux CAN Tx"
  Accu CAN Tx/1 -> Bus Creator/3, Data Type Conversion2/1  "Accu CAN Tx"
  Torque CAN Tx/1 -> Bus Creator/4, Data Type Conversion3/1  "Torque CAN Tx"
  CAN Channels Status/1 -> Bus Creator/5, Data Type Conversion4/1  "CAN Channels Status"
  Dash CAN Rx/1 -> Bus Creator/6, Data Type Conversion5/1  "Dash CAN Rx"
  Aux CAN Rx/1 -> Bus Creator/7, Data Type Conversion6/1  "Aux CAN Rx"
  Accu CAN Rx/1 -> Bus Creator/8, Data Type Conversion7/1  "Accu CAN Rx"
  Inv LEFT CAN Rx/1 -> Bus Creator/9, Data Type Conversion8/1  "Inv LEFT CAN Rx"
  Inv RIGHT CAN Rx/1 -> Bus Creator/10, Data Type Conversion9/1  "Inv RIGHT CAN Rx"
  "Sensor Error OR "/1 -> Bus Creator1/1, Data Type Conversion10/1  "Sensor Error"
  Plausibility OR/1 -> Bus Creator1/2, Data Type Conversion11/1  "Plausibility"
  Safe State OR/1 -> Bus Creator1/4, Data Type Conversion13/1  "TSAL Safe State"
  BMS Status OR/1 -> Bus Creator1/5, Data Type Conversion14/1  "BMS Status"
  Bus Creator/1 -> Bus Creator2/1  "CAN States"
  Bus Creator1/1 -> Bus Creator2/3  "Systems States"
  Bus Creator2/1 -> Bus Selector5/1
  Bus Selector5/1 -> Enable AND/1  "<Dash CAN Tx>"
  Bus Selector5/2 -> Enable AND/2  "<Aux CAN Tx>"
  Bus Selector5/3 -> Enable AND/3  "<Accu CAN Tx>"
  Bus Selector5/4 -> Enable AND/4  "<Torque CAN Tx>"
  Bus Selector5/5 -> Enable AND/5  "<CAN Channels Status>"
  Bus Selector5/6 -> Enable AND/6  "<Dash CAN Rx>"
  Bus Selector5/7 -> Enable AND/7  "<Aux CAN Rx>"
  Bus Selector5/8 -> Enable AND/8  "<Accu CAN Rx>"
  Bus Selector5/9 -> Enable AND/9  "<Inv LEFT CAN Rx>"
  Bus Selector5/10 -> Enable AND/10  "<Inv RIGHT CAN Rx>"
  Bus Selector5/11 -> Enable AND/11  "<Start Up Proc>"
  Bus Selector5/12 -> Enable AND/12  "<Sensor Error>"
  Bus Selector5/13 -> Enable AND/13  "<Plausibility>"
  Bus Selector5/14 -> Enable AND/14  "<BSPD State>"
  Bus Selector5/15 -> Enable AND/15  "<TSAL Safe State>"
  Bus Selector5/16 -> Enable AND/16  "<BMS Status>"
  Logical Operator15/1 -> Buzzer Set/1, Resettable Delay 1.5s/2, Resettable Delay 1.5s/1
  Enable AND/1 -> Logical Operator15/1
  Constant12/1 -> Logical Operator16/1
  Logical Operator16/1 -> Logical Operator15/2
  BSPD OR/1 -> Bus Creator1/3, Data Type Conversion12/1  "BSPD State"
  Logical Operator/1 -> "Sensor Error OR "/1
  Logical Operator1/1 -> Plausibility OR/1
  to 100Hz16/1 -> BSPD OR/1  "BSPD State"
  Constant11/1 -> BSPD OR/2
  Data Type Conversion/1 -> USB_FLIGHT_REC_BL3/1
  Data Type Conversion1/1 -> USB_FLIGHT_REC_BL4/1
  Data Type Conversion2/1 -> USB_FLIGHT_REC_BL5/1
  Data Type Conversion3/1 -> USB_FLIGHT_REC_BL6/1
  Data Type Conversion4/1 -> USB_FLIGHT_REC_BL7/1
  Data Type Conversion5/1 -> USB_FLIGHT_REC_BL8/1
  Data Type Conversion6/1 -> USB_FLIGHT_REC_BL9/1
  Data Type Conversion7/1 -> USB_FLIGHT_REC_BL10/1
  Data Type Conversion8/1 -> USB_FLIGHT_REC_BL11/1
  Data Type Conversion9/1 -> USB_FLIGHT_REC_BL12/1
  Data Type Conversion10/1 -> USB_FLIGHT_REC_BL13/1
  Data Type Conversion11/1 -> USB_FLIGHT_REC_BL14/1
  Data Type Conversion12/1 -> USB_FLIGHT_REC_BL15/1
  Data Type Conversion13/1 -> USB_FLIGHT_REC_BL16/1
  Data Type Conversion14/1 -> USB_FLIGHT_REC_BL17/1
  Logical Operator2/1 -> Safe State OR/1
  Logical Operator3/1 -> BMS Status OR/1
  Logical Operator10/1 -> Dash CAN Tx/1, Aux CAN Tx/1, Accu CAN Tx/1, Torque CAN Tx/1
  Logical Operator11/1 -> Dash CAN Rx/1, Aux CAN Rx/1, Accu CAN Rx/1, Inv RIGHT CAN Rx/1, Inv LEFT CAN Rx/1
